simulink model "viatura"  (R2015a)
settings: Solver=ode45  StartTime=0.0  StopTime=tsim  RelTol=1e-3
values from neighbouring files (symbols this model uses):
  beta = 5    [lab1.m]
  m = 1    [lab1.m]
  v0 = ',num2str(v0),'m/s'])    [lab1.m]
settings Model: Creator=Alunos  LastModifiedBy=Diogo

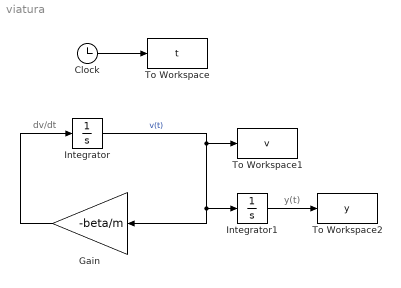
== system viatura ==
  note: y(t)
  note: dv/dt
  Clock : Clock
  Gain : Gain  Gain=-beta/m
  Integrator : Integrator  InitialCondition=v0
  Integrator1 : Integrator
  To Workspace : ToWorkspace  VariableName=t  SampleTime=-1
  To Workspace1 : ToWorkspace  VariableName=v  SampleTime=-1
  To Workspace2 : ToWorkspace  VariableName=y  SampleTime=-1
  wires:
  Gain/1 -> Integrator/1
  Clock/1 -> To Workspace/1
  Integrator/1 -> To Workspace1/1, Gain/1, Integrator1/1  "v(t)"
  Integrator1/1 -> To Workspace2/1
